simulink model "MosquittoPqth"  (R2019b)
settings: Solver=FixedStepAuto  StartTime=0.0  StopTime=60  FixedStep=0.01  RelTol=1e-3
libraries: simulink x5, simulink_extras x2
settings Model: Creator=killidaen  LastModifiedBy=killidaen
settings SFSimCC: CustomCodeUndefinedFunction=UseInterfaceOnly

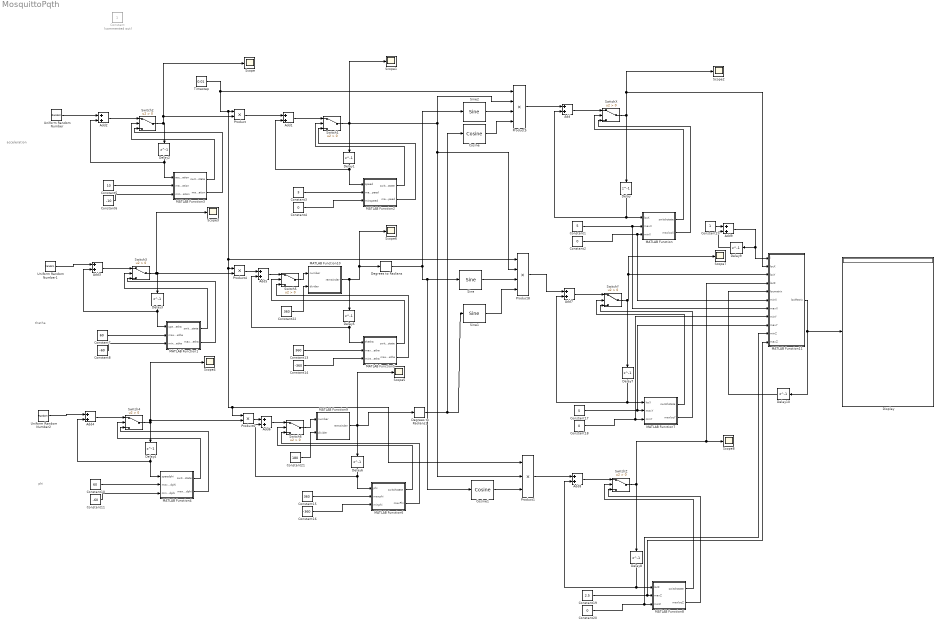
== system MosquittoPqth ==
  note: phi
  note: thetha
  note: acceleration
  Add{,1..9} (10 alike) : Sum
  Constant : Constant  Commented=on
  Constant1 : Constant  Value=5
  Constant10 : Constant  Value=60
  Constant11 : Constant  Value=-60
  Constant13 : Constant  Value=360
  Constant14 : Constant  Value=-360
  Constant15 : Constant  Value=360
  Constant16 : Constant  Value=-360
  Constant17 : Constant  Value=5
  Constant{2,4,18,20} (4 alike) : Constant  Value=0
  Constant19 : Constant  Value=2.5
  Constant21 : Constant  Value=180
  Constant22 : Constant  Value=360
  Constant23 : Constant
  Constant3 : Constant  Value=3
  Constant5 : Constant  Value=10
  Constant6 : Constant  Value=-10
  Constant7 : Constant  Value=60
  Constant8 : Constant  Value=-60
  Cosine : simulink/Lookup Tables/Cosine  Formula=cos(2*pi*u)  NumDataPoints=(2^5)+1  OutputWordLength=16  InternalRulePriority=Speed
      settings: SourceProductName=Simulink  SourceProductBaseCode=SL
  Cosine1 : simulink/Lookup Tables/Cosine  Formula=cos(2*pi*u)  NumDataPoints=(2^5)+1  OutputWordLength=16  InternalRulePriority=Speed
      settings: SourceProductName=Simulink  SourceProductBaseCode=SL
  Degrees to Radians : simulink_extras/Transformations/Degrees to Radians
  Degrees to Radians1 : simulink_extras/Transformations/Degrees to Radians
  Delay : Delay  DelayLength=1  InitialCondition=5
  Delay{1..6,9..10} (8 alike) : Delay  DelayLength=1  InitialCondition=0
  Delay7 : Delay  DelayLength=1  InitialCondition=5
  Delay8 : Delay  DelayLength=1  InitialCondition=2.5
  Display : Display
  MATLAB Function : MATLAB Function  TreatAsAtomicUnit=on
  MATLAB Function1 : MATLAB Function  TreatAsAtomicUnit=on
  MATLAB Function10 : MATLAB Function  TreatAsAtomicUnit=on
  MATLAB Function11 : MATLAB Function  TreatAsAtomicUnit=on
  MATLAB Function2 : MATLAB Function  TreatAsAtomicUnit=on
  MATLAB Function3 : MATLAB Function  TreatAsAtomicUnit=on
  MATLAB Function4 : MATLAB Function  TreatAsAtomicUnit=on
  MATLAB Function5 : MATLAB Function  TreatAsAtomicUnit=on
  MATLAB Function6 : MATLAB Function  TreatAsAtomicUnit=on
  MATLAB Function7 : MATLAB Function  TreatAsAtomicUnit=on
  MATLAB Function8 : MATLAB Function  TreatAsAtomicUnit=on
  MATLAB Function9 : MATLAB Function  TreatAsAtomicUnit=on
  Product : Product
  Product1 : Product  Inputs=3
  Product4 : Product
  Product5 : Product  Inputs=4
  Product6 : Product
  Product8 : Product  Inputs=4
  Scope{,1..8} (9 alike) : Scope
  Sine : simulink/Lookup Tables/Sine  Formula=sin(2*pi*u)  NumDataPoints=(2^5)+1  OutputWordLength=16  InternalRulePriority=Speed
      settings: SourceProductName=Simulink
  Sine1 : simulink/Lookup Tables/Sine  Formula=sin(2*pi*u)  NumDataPoints=(2^5)+1  OutputWordLength=16  InternalRulePriority=Speed
      settings: SourceProductName=Simulink
  Sine2 : simulink/Lookup Tables/Sine  Formula=sin(2*pi*u)  NumDataPoints=(2^5)+1  OutputWordLength=16  InternalRulePriority=Speed
      settings: SourceProductName=Simulink
  Switch{1..6} (6 alike) : Switch  Criteria=u2 > Threshold
  SwitchX : Switch  Criteria=u2 > Threshold
  SwitchY : Switch  Criteria=u2 > Threshold
  SwitchZ : Switch  Criteria=u2 > Threshold
  Timestep : Constant  Value=0.01
  Uniform Random Number : UniformRandomNumber  Minimum=-5  Maximum=5  Seed=142  SampleTime=0.01
  Uniform Random Number1 : UniformRandomNumber  Minimum=-15  Maximum=15  Seed=95  SampleTime=0.01
  Uniform Random Number2 : UniformRandomNumber  Minimum=-15  Maximum=15  Seed=36  SampleTime=0.01
  wires:
  Add/1 -> SwitchX/1
  MATLAB Function/1(switchstate) -> SwitchX/2
  MATLAB Function/2(maxlocX) -> SwitchX/3
  Constant1/1 -> MATLAB Function11/7(maxX), MATLAB Function/2(maxX)
  Constant2/1 -> MATLAB Function11/6(minX), MATLAB Function/3(minX)
  Constant4/1 -> MATLAB Function2/3(minspeed)
  MATLAB Function2/2(maxSpeed) -> Switch1/3
  Constant3/1 -> MATLAB Function2/2(maxspeed)
  Add1/1 -> Switch1/1
  Switch1/1 -> Product5/2, Product1/2, Product8/2, Scope1/1, Delay1/1
  MATLAB Function2/1(switchstate) -> Switch1/2
  MATLAB Function3/1(switchstate) -> Switch2/2
  Add2/1 -> Switch2/1
  Constant5/1 -> MATLAB Function3/2(maxacceleration)
  Constant6/1 -> MATLAB Function3/3(minacceleration)
  MATLAB Function3/2(maxAcceleration) -> Switch2/3
  Uniform Random Number/1 -> Add2/1
  Product/1 -> Add1/1
  Product5/1 -> Add/1
  Delay1/1 -> Add1/2, MATLAB Function2/1(speed)
  Delay/1 -> MATLAB Function/1(locX), Add/2
  Switch2/1 -> Delay2/1, Scope/1, Product/2
  Delay2/1 -> Add2/2, MATLAB Function3/1(acceleration)
  MATLAB Function1/2(maxSpeedthetha) -> Switch3/3
  Constant8/1 -> MATLAB Function1/3(minspeedthetha)
  Constant7/1 -> MATLAB Function1/2(maxspeedthetha)
  Add3/1 -> Switch3/1
  MATLAB Function1/1(switchstate) -> Switch3/2
  Delay3/1 -> Add3/2, MATLAB Function1/1(speedthetha)
  Uniform Random Number1/1 -> Add3/1
  Delay4/1 -> Add4/2, MATLAB Function4/1(speedphi)
  Add4/1 -> Switch4/1
  Constant11/1 -> MATLAB Function4/3(minspeedphi)
  Uniform Random Number2/1 -> Add4/1
  MATLAB Function4/1(switchstate) -> Switch4/2
  Switch4/1 -> Delay4/1, Scope4/1, Product6/2
  MATLAB Function4/2(maxSpeedphi) -> Switch4/3
  Constant10/1 -> MATLAB Function4/2(maxspeedphi)
  Product4/1 -> Add5/1
  MATLAB Function5/1(switchstate) -> Switch5/2
  Constant14/1 -> MATLAB Function5/3(minthetha)
  MATLAB Function5/2(maxThetha) -> Switch5/3
  Add5/1 -> Switch5/1
  Delay5/1 -> Add5/2, MATLAB Function5/1(thetha)
  Switch3/1 -> Scope3/1, Delay3/1, Product4/2
  Constant13/1 -> MATLAB Function5/2(maxthetha)
  MATLAB Function6/2(maxPhi) -> Switch6/3
  Add6/1 -> Switch6/1
  Constant15/1 -> MATLAB Function6/2(maxphi)
  Delay6/1 -> Add6/2, MATLAB Function6/1(phi)
  MATLAB Function6/1(switchstate) -> Switch6/2
  Constant16/1 -> MATLAB Function6/3(minphi)
  Product6/1 -> Add6/1
  Timestep/1 -> Product8/1, Product1/1, Product6/1, Product4/1, Product/1, Product5/1
  Constant18/1 -> MATLAB Function7/3(minY), MATLAB Function11/8(minY)
  MATLAB Function7/2(maxlocY) -> SwitchY/3
  Add7/1 -> SwitchY/1
  SwitchY/1 -> Scope7/1, MATLAB Function11/3(locY), Delay7/1
  MATLAB Function7/1(switchstate) -> SwitchY/2
  Delay7/1 -> MATLAB Function7/1(locY), Add7/2
  Product8/1 -> Add7/1
  Constant17/1 -> MATLAB Function11/9(maxY), MATLAB Function7/2(maxY)
  MATLAB Function8/1(switchstate) -> SwitchZ/2
  Constant19/1 -> MATLAB Function11/11(maxZ), MATLAB Function8/2(maxZ)
  Product1/1 -> Add8/1
  Add8/1 -> SwitchZ/1
  SwitchZ/1 -> MATLAB Function11/4(locZ), Scope8/1, Delay8/1
  MATLAB Function8/2(maxlocZ) -> SwitchZ/3
  Constant20/1 -> MATLAB Function11/10(minZ), MATLAB Function8/3(minZ)
  Delay8/1 -> MATLAB Function8/1(locZ), Add8/2
  Degrees to Radians/1 -> Sine2/1, Sine/1, Cosine1/1
  Sine/1 -> Product8/3
  Degrees to Radians1/1 -> Cosine/1, Sine1/1
  Sine1/1 -> Product8/4
  Sine2/1 -> Product5/3
  Cosine/1 -> Product5/4
  Cosine1/1 -> Product1/3
  MATLAB Function9/1(remainder) -> Scope5/1, Delay6/1, Degrees to Radians1/1
  Switch6/1 -> MATLAB Function9/1(number)
  Constant21/1 -> MATLAB Function9/2(divider)
  MATLAB Function10/1(remainder) -> Scope6/1, Degrees to Radians/1, Delay5/1
  Switch5/1 -> MATLAB Function10/1(number)
  Constant22/1 -> MATLAB Function10/2(divider)
  Add9/1 -> MATLAB Function11/1(i), Delay9/1
  SwitchX/1 -> MATLAB Function11/2(locX), Scope2/1, Delay/1
  MATLAB Function11/1(locMatrix) -> Delay10/1, Display/1
  Constant23/1 -> Add9/1
  Delay9/1 -> Add9/2
  Delay10/1 -> MATLAB Function11/5(locmatrix)

== matlab function MosquittoPqth/MATLAB Function2 ==
  data: speed input; switchstate output; maxspeed input; maxSpeed output; minspeed input
function [switchstate,maxSpeed]= fcn(speed, maxspeed, minspeed)

    if (speed > maxspeed)
        maxSpeed = maxspeed;
        switchstate = 0;
    elseif (speed < minspeed)
        maxSpeed = minspeed;
        switchstate = 0;
    else
        maxSpeed = speed;
        switchstate = 1;
    end

== matlab function MosquittoPqth/MATLAB Function ==
  data: locX input; switchstate output; maxX input; maxlocX output; minX input
function [switchstate,maxlocX]= fcn(locX, maxX, minX)

    if (locX > maxX)
        maxlocX = maxX;
        switchstate = 0;
    elseif (locX < minX)
        maxlocX = minX;
        switchstate = 0;
    else
        maxlocX = locX;
        switchstate = 1;
    end

== matlab function MosquittoPqth/MATLAB Function3 ==
  data: acceleration input; switchstate output; maxacceleration input; maxAcceleration output; minacceleration input
function [switchstate,maxAcceleration]= fcn(acceleration, maxacceleration, minacceleration)
    if (acceleration > maxacceleration)
        maxAcceleration = maxacceleration;
        switchstate = 0;
    elseif (acceleration < minacceleration)
        maxAcceleration = minacceleration;
        switchstate = 0;
    else
        maxAcceleration = acceleration;
        switchstate = 1;
    end

== matlab function MosquittoPqth/MATLAB Function1 ==
  data: speedthetha input; switchstate output; maxspeedthetha input; maxSpeedthetha output; minspeedthetha input
function [switchstate,maxSpeedthetha]= fcn(speedthetha, maxspeedthetha, minspeedthetha)
    if (speedthetha > maxspeedthetha)
        maxSpeedthetha = maxspeedthetha;
        switchstate = 0;
    elseif (speedthetha < minspeedthetha)
        maxSpeedthetha = minspeedthetha;
        switchstate = 0;
    else
        maxSpeedthetha = speedthetha;
        switchstate = 1;
    end

== matlab function MosquittoPqth/MATLAB Function4 ==
  data: speedphi input; switchstate output; maxspeedphi input; maxSpeedphi output; minspeedphi input
function [switchstate,maxSpeedphi]= fcn(speedphi, maxspeedphi, minspeedphi)
    if (speedphi > maxspeedphi)
        maxSpeedphi = maxspeedphi;
        switchstate = 0;
    elseif (speedphi < minspeedphi)
        maxSpeedphi = minspeedphi;
        switchstate = 0;
    else
        maxSpeedphi = speedphi;
        switchstate = 1;
    end

== matlab function MosquittoPqth/MATLAB Function5 ==
  data: thetha input; switchstate output; maxthetha input; maxThetha output; minthetha input
function [switchstate,maxThetha]= fcn(thetha, maxthetha, minthetha)

    if (thetha > maxthetha)
        maxThetha = maxthetha;
        switchstate = 0;
    elseif (thetha < minthetha)
        maxThetha = minthetha;
        switchstate = 0;
    else
        maxThetha = thetha;
        switchstate = 1;
    end

== matlab function MosquittoPqth/MATLAB Function6 ==
  data: phi input; switchstate output; maxphi input; maxPhi output; minphi input
function [switchstate,maxPhi]= fcn(phi, maxphi, minphi)

    if (phi > maxphi)
        maxPhi = maxphi;
        switchstate = 0;
    elseif (phi < minphi)
        maxPhi = minphi;
        switchstate = 0;
    else
        maxPhi = phi;
        switchstate = 1;
    end

== matlab function MosquittoPqth/MATLAB Function7 ==
  data: locY input; switchstate output; maxY input; maxlocY output; minY input
function [switchstate,maxlocY]= fcn(locY, maxY, minY)

    if (locY > maxY)
        maxlocY = maxY;
        switchstate = 0;
    elseif (locY < minY)
        maxlocY = minY;
        switchstate = 0;
    else
        maxlocY = locY;
        switchstate = 1;
    end

== matlab function MosquittoPqth/MATLAB Function8 ==
  data: locZ input; switchstate output; maxZ input; maxlocZ output; minZ input
function [switchstate,maxlocZ]= fcn(locZ, maxZ, minZ)

    if (locZ > maxZ)
        maxlocZ = maxZ;
        switchstate = 0;
    elseif (locZ < minZ)
        maxlocZ = minZ;
        switchstate = 0;
    else
        maxlocZ = locZ;
        switchstate = 1;
    end

== matlab function MosquittoPqth/MATLAB Function9 ==
  data: number input; remainder output; divider input
function remainder = fcn(number,divider)

    remainder = rem(number,divider);

== matlab function MosquittoPqth/MATLAB Function10 ==
  data: number input; remainder output; divider input
function remainder = fcn(number,divider)

    remainder = rem(number,divider);

== matlab function MosquittoPqth/MATLAB Function11 ==
  data: i input; locX input; locY input; locMatrix output; locZ input; locmatrix input; minX input; maxX input; minY input; maxY input; minZ input; maxZ input
function locMatrix = fcn(i,locX,locY,locZ, locmatrix,minX,maxX,minY,maxY,minZ,maxZ)
   locMatrix = zeros(1,3);
   if (locX < minX)
       locX = minX;
   elseif (locX > maxX)
       locX = maxX;
   else
   end
   locMatrix(1,1) = locX;
   
   if (locY < minY)
       locY = minY;
   elseif (locY > maxY)
       locY = maxY;
   else
   end
   locMatrix(1,2) = locY;
   
   if (locZ < minZ)
       locZ = minZ;
   elseif (locZ > maxZ)
       locZ = maxZ;
   else
   end
   locMatrix(1,3) = locZ;
